simulink model "InnerOuter_Sim_newNav"  (Simulink 7.8)
settings: Solver=ode4  StartTime=0.0  StopTime=300  FixedStep=SampleT  RelTol=1e-3
InitFcn:
  | clc
  | innerOuterInit
values from neighbouring files (symbols this model uses):
  apSampleTime = 0.01    [innerOuterInit.m]
  SampleT = 0.005    [innerOuterInit.m]
  T = 0.01    [innerOuterInit.m]
undefined symbols (not defined in the file or in its folder): A1, Apolar, baseHeight, BasePoint, baseTemp, CD0, chord, CL0, CLa, CLa_dot, Clb, ClDa, CLDe, CLDf, ClDr, clock, Clp, CLq, Clr, Cm0, Cma, CmDe, CmDf, Cmq, Cnb, CnDa, CnDr, Cnp, Cnr, compensatorOn, CYb, CYDr, da_failamp, da_failbias, da_failper, daL_fail, daR_fail, deg, DiscIntNeverNeededParam, dr_fail, dr_failamp, dr_failbias, dr_failper, Earth, elarm, Euler_0, F, gaind, Init_onlyOnce, Init_Reset, ISA_g, Ixx, Iyy, Izz, L1OF, lapseRate, Light, mass, MIL, MinThK ... (+21)
libraries: simulink x69, aerolibconvert2 x19, SLUGS_Library x10, aerolibactuator x5, aerolibobsolete x3, dspmtrx3 x3, aerolibwind2 x2, aerolibtransform2 x1, aerolibatmos2 x1, dsPICdrivers x1
(part 1 of 3)
CloseFcn:
  | rtwprivate ssgencode ModelCloseRequest AttitudeComplementary
settings Model: Creator=ASL_Lab  LastModifiedBy=User  BufferReuse=off
settings OptimizationCC: BlockReduction=off  ConditionallyExecuteInputs=off  OptimizeBlockIOStorage=off  BufferReuse=off  ExpressionFolding=off  LocalBlockOutputs=off  InitFltsAndDblsToZero=on
settings DebuggingCC: ConsistencyChecking=warning  AlgebraicLoopMsg=error  SaveWithParameterizedLinksMsg=none  MultiTaskDSMMsg=warning  MultiTaskCondExecSysMsg=none  FcnCallInpInsideContextMsg=Use local settings  ModelReferenceExtraNoncontSigs=warning  StrictBusMsg=None
settings HardwareCC: TargetHWDeviceType=32-bit Generic
settings SFSimCC: SimParseCustomCode=off
settings RTWCC: IncludeERTFirstTime=on
settings GRTTargetCC: TargetFcnLib=ansi_tfl_tmw.mat

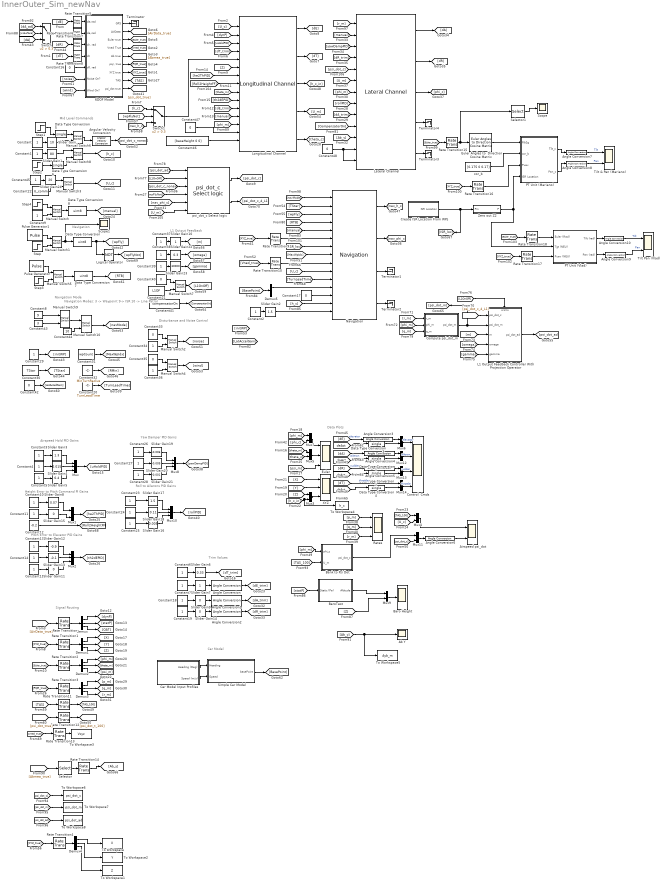
== system InnerOuter_Sim_newNav ==
  note: Mid Level Commands
  note: Trim Values
  note: Signal Routing
  note: Airspeed Hold PID Gains
  note: Height Error to Pitch Command PI Gains
  note: Pitch Error to Elevator PID Gains
  note: Data Plots
  note: Yaw Damper PID Gains
  note: Roll to Ailerons PID Gains
  note: Navigation
  note: Disturbance and Noise Control
  note: L1 Output Feedback
  note: Car Model
  note: Navigation Mode
  note: Navigation Modes:
      | 3 -> Waypoint
      | 9-> ISR
      | 10 -> Line Patrol
  6DOF Model : Subsystem
  Ab Y : Scope
      settings: TimeRange=140  YMin=-3  YMax=3  SaveName=ScopeData9
  Airspeed psi_dot : Scope  NumInputPorts=2
      settings: TimeRange=125  YMin=14.91~-37.5  YMax=15.05~5  SaveName=AirspeedPsiDot
  Angle Conversion : aerolibconvert2/Angle Conversion  IU=deg  OU=rad
  Angle Conversion1 : aerolibconvert2/Angle Conversion  IU=deg  OU=rad
  Angle Conversion{3..10} (8 alike) : aerolibconvert2/Angle Conversion  IU=rad  OU=deg
  Angle Conversion2 : aerolibconvert2/Angle Conversion  IU=deg  OU=rad
  Angular Velocity Conversion : aerolibconvert2/Angular Velocity Conversion  IU=deg/s  OU=rad/s
  Bank to Psi Dot : Subsystem  AncestorBlock=SLUGS_Library/Navigation/Bank to Psi Dot
  Baro Height : Scope
      settings: TimeRange=350  YMin=-1500  YMax=700  SaveName=AirspeedPsiDot1
  BaroTest : Subsystem
  Car Model Input Profiles : Subsystem  Tag=STV Subsys  LoadFcn=sigbuilder_block('load');  StartFcn=sigbuilder_block('start');  StopFcn=sigbuilder_block('stop');  ClipboardFcn=sigbuilder_block('clipboard');  mask(Sigbuilder block){}
      mask help: Sigbuilder GUI
      mask init:
      | if ~strcmp(get_param(bdroot(gcbh),'SimulationStatus'),'stopped') tuvar = sigbuilder_block('maskInit'); end
      settings: CopyFcn=sigbuilder_block('copy');  DeleteFcn=sigbuilder_block('delete');  ModelCloseFcn=sigbuilder_block('modelClose');  PreSaveFcn=sigbuilder_block('preSave');  NameChangeFcn=sigbuilder_block('namechange');  OpenFcn=sigbuilder_block('open',[437.25 199.5 550.5 399.75 ]);  CloseFcn=sigbuilder_block('close');
      mask Display: plot(0,0,100,100,[10,10,40,40,10],[80,20,20,80,80],[40,10],[50,50], [40,27,10],[65,72,56],[40,25,25,10],[28,28,43,43]);
  Compute psi_dot_m : Subsystem
  Constant{,1..7,10..11,13..15,18..19,23..28,37..39,45} (25 alike) : Constant  OutDataTypeStr=single  SampleTime=apSampleTime
  Constant12 : Constant  Value=-0.2  OutDataTypeStr=single  SampleTime=apSampleTime
  Constant16 : Constant  Value=0
  Constant{17,40,47..48} (4 alike) : Constant  Value=0  OutDataTypeStr=uint8  SampleTime=apSampleTime
  Constant20 : Constant  Value=TurnLeadTime  SampleTime=apSampleTime
  Constant21 : Constant  Value=L1OF  OutDataTypeStr=single  SampleTime=apSampleTime
  Constant22 : Constant  Value=U_comm  SampleTime=apSampleTime
  Constant29 : Constant  OutDataTypeStr=uint8  SampleTime=apSampleTime
  Constant30 : Constant  Value=TStar  OutDataTypeStr=single  SampleTime=apSampleTime
  Constant31 : Constant  Value=wpCount  OutDataTypeStr=uint8  SampleTime=apSampleTime
  Constant32 : Constant  Value=MinTurnRadius  SampleTime=apSampleTime
  Constant33 : Constant  Value=0  SampleTime=SampleT
  Constant34 : Constant  SampleTime=SampleT
  Constant35 : Constant  Value=0  SampleTime=SampleT
  Constant36 : Constant  SampleTime=SampleT
  Constant41 : Constant  Value=compensatorOn  SampleTime=apSampleTime
  Constant42 : Constant  Value=0  SampleTime=apSampleTime
  Constant43 : Constant  Value=3  OutDataTypeStr=uint8  SampleTime=apSampleTime
  Constant44 : Constant  Value=10  OutDataTypeStr=uint8  SampleTime=apSampleTime
  Constant46 : Constant  Value=[baseHeight 0 0]  OutDataTypeStr=single
  Constant8 : Constant  Value=9  OutDataTypeStr=uint8  SampleTime=apSampleTime
  Constant9 : Constant  OutDataTypeStr=uint8  SampleTime=apSampleTime
  Control  Cmds : Scope  NumInputPorts=4
      settings: TickLabels=on  TimeRange=100  YMin=-2~-10~-11~0.225  YMax=3.5~17.5~1~0.425  SaveName=ctrlCmds
  Create ISR Location From WPs : Subsystem
  Data Type Conversion : DataTypeConversion  OutDataTypeStr=uint8
  Data Type Conversion{1..6} (6 alike) : DataTypeConversion  OutDataTypeStr=single
  Data Type Conversion7 : DataTypeConversion  OutDataTypeStr=uint8
  Data Type Conversion8 : DataTypeConversion  OutDataTypeStr=uint8
  Demux{,1..4} (5 alike) : Demux  Outputs=3
  Demux5 : Demux  Outputs=[2 1]
  Euler : Scope  NumInputPorts=3
      settings: TimeRange=100  YMin=-0.4~-0.02~0  YMax=1~0.06~7  SaveName=EulerData  DataFormat=Structure
  Euler Angles to  Direction Cosine Matrix : aerolibobsolete/Euler Angles to  Direction Cosine Matrix
  L1 Output Feedback Controller With  Projection Operator : Subsystem  TreatAsAtomicUnit=on
  Lateral Channel : SLUGS_Library/Control Blocks/Lateral Channel
  Logical Operator : Logic  Operator=NOT  AllPortsSameDT=off  OutDataTypeStr=boolean
  Longitudinal Channel : SLUGS_Library/Control Blocks/Longitudinal Channel
  Manual Switch{,2,4,7..8,10} (6 alike) : simulink/Signal Routing/Manual Switch  sw=1  action=0  varsize=off
  Manual Switch{1,3,5..6,9} (5 alike) : simulink/Signal Routing/Manual Switch  sw=0  action=0  varsize=off
  Mux{,2,8,10} (4 alike) : Mux  Inputs=3
  Mux{1,3..7,9,11..14} (11 alike) : Mux  Inputs=2
  Navigation : SLUGS_Library/Navigation/Navigation
  PT Unit (Mariano) : Subsystem  TreatAsAtomicUnit=on  SystemSampleTime=0.01
  "PT Unit (Vlad) " : Subsystem
  Pulse Generator : DiscretePulseGenerator  Period=200*100  PulseWidth=30*100  PhaseDelay=120*100  SampleTime=0.01
  Pulse Generator1 : DiscretePulseGenerator  Period=70*100  PulseWidth=45*100  PhaseDelay=0*100  SampleTime=0.01
  Rate Transition{,1..4,9..18} (15 alike) : RateTransition  OutPortSampleTime=apSampleTime
  Rate Transition{5..8} (4 alike) : RateTransition  OutPortSampleTime=SampleT
  Rates : Scope  NumInputPorts=3
      settings: TimeRange=300  YMin=-0.75~-1.5~-0.3  YMax=1~1.5~0.7  SaveName=ScopeData3
  Scope : Scope
      settings: YMin=5.2  YMax=6.3  SaveName=ScopeData2
  Scope1 : Scope
      settings: TimeRange=400  YMin=0.95  YMax=1.05  SaveName=ScopeData10
  Selector : Selector  InputPortWidth=3  IndexOptions=Index vector (dialog)  Indices=[2]  OutputSizes=1
  Selector1 : Selector  InputPortWidth=3  IndexOptions=Index vector (dialog)  Indices=[3]  OutputSizes=1
  Simple Car Model : Subsystem
  Slider Gain : simulink/Math Operations/Slider Gain  low=-18  gain=10  high=18
  Slider Gain1 : simulink/Math Operations/Slider Gain  low=0  gain=80  high=800
  Slider Gain10 : simulink/Math Operations/Slider Gain  low=0  gain=1  high=10
  Slider Gain11 : simulink/Math Operations/Slider Gain  low=-0.1  gain=0  high=0
  Slider Gain12 : simulink/Math Operations/Slider Gain  low=-2  gain=-0.9  high=0.3
  Slider Gain13 : simulink/Math Operations/Slider Gain  low=-0.1  gain=-0.1  high=0
  Slider Gain14 : simulink/Math Operations/Slider Gain  low=-10  gain=0  high=10
  Slider Gain15 : simulink/Math Operations/Slider Gain  low=-20  gain=0  high=20
  Slider Gain16 : simulink/Math Operations/Slider Gain  low=-0.1  gain=0.005  high=0.1
  Slider Gain17 : simulink/Math Operations/Slider Gain  low=-0.1  gain=1.5  high=5
  Slider Gain18 : simulink/Math Operations/Slider Gain  low=0  gain=0.11  high=2
  Slider Gain19 : simulink/Math Operations/Slider Gain  low=-20  gain=-0.006  high=20
  Slider Gain2 : simulink/Math Operations/Slider Gain  low=0  gain=1.5  high=2
  Slider Gain20 : simulink/Math Operations/Slider Gain  low=-20  gain=-0.009  high=20
  Slider Gain21 : simulink/Math Operations/Slider Gain  low=-20  gain=-0.001  high=20
  Slider Gain22 : simulink/Math Operations/Slider Gain  low=0  gain=0.3  high=5
  Slider Gain23 : simulink/Math Operations/Slider Gain  low=-50000  gain=30000  high=50000
  Slider Gain24 : simulink/Math Operations/Slider Gain  low=0  gain=20  high=50
  Slider Gain3 : simulink/Math Operations/Slider Gain  low=0  gain=1.3  high=4.5
  Slider Gain4 : simulink/Math Operations/Slider Gain  low=-20  gain=0.015  high=20
  Slider Gain5 : simulink/Math Operations/Slider Gain  low=-20  gain=0.4  high=20
  Slider Gain6 : simulink/Math Operations/Slider Gain  low=0.1  gain=0.33  high=1
  Slider Gain7 : simulink/Math Operations/Slider Gain  low=-10  gain=1  high=10
  Slider Gain8 : simulink/Math Operations/Slider Gain  low=-20  gain=0.07  high=20
  Slider Gain9 : simulink/Math Operations/Slider Gain  low=-10  gain=0  high=10
  Step : Step  Time=0.01  SampleTime=0.01
  Step1 : Step  Time=10  After=5  SampleTime=0.01
  Step2 : Step  Time=10  Before=Pos_0(3)  After=500  SampleTime=0.01
  Step3 : Step  Time=1500  SampleTime=0.01
  Step4 : Step  Time=0.01  Before=1  After=0  SampleTime=0.01
  Switch : Switch  Criteria=u2 > Threshold  Threshold=0.3  OutDataTypeStr=Inherit: Inherit via back propagation  SampleTime=apSampleTime  InputSameDT=on
  Switch1 : Switch  Criteria=u2 > Threshold  Threshold=0.3  OutDataTypeStr=Inherit: Inherit via back propagation  InputSameDT=on
  Terminator{,1..4} (5 alike) : Terminator
  Tilt & Pan (Mariano) : Scope  NumInputPorts=2
      settings: TimeRange=125  YMin=60~-90  YMax=90~90  SaveName=AirspeedPsiDot2
  Tilt Pan (Vlad) : Scope  NumInputPorts=2
      settings: TimeRange=125  YMin=-100~-90  YMax=100~-50  SaveName=AirspeedPsiDot3
  To Workspace : ToWorkspace  VariableName=X  SampleTime=-1  SaveFormat=Array
  To Workspace1 : ToWorkspace  VariableName=Z  SampleTime=-1  SaveFormat=Array
  To Workspace2 : ToWorkspace  VariableName=Y  SampleTime=-1  SaveFormat=Array
  To Workspace3 : ToWorkspace  VariableName=Vxyz  SampleTime=-1  SaveFormat=Array
  To Workspace4 : ToWorkspace  VariableName=h_c  SampleTime=-1  SaveFormat=Array
  To Workspace5 : ToWorkspace  VariableName=Ayb_m  SampleTime=.01  SaveFormat=Array
  To Workspace6 : ToWorkspace  VariableName=psi_dot_c  SampleTime=.01  SaveFormat=Array
  To Workspace7 : ToWorkspace  VariableName=psi_dot_m  SampleTime=.01  SaveFormat=Array
  To Workspace8 : ToWorkspace  VariableName=psi_dot_ad  SampleTime=.01  SaveFormat=Array
  XYZ : Scope  NumInputPorts=3
      settings: TimeRange=125  YMin=-250~-200~180  YMax=100~200~230
  Zero out Z2 : MATLAB Function  TreatAsAtomicUnit=on
  cor_b : Constant  Value=[0.175 0 0.17]  OutDataTypeStr=single
  psi_dot_c Select logic : SLUGS_Library/Control Blocks/psi_dot_c Select logic
  wires:
  6DOF Model/7(XYZ true) -> [XYZ_true]
  6DOF Model/4(Vned True) -> [Vned_true]
  6DOF Model/5(Ab true) -> [Abmea_true]
  6DOF Model/6("pqr, true") -> [PQR_true]
  6DOF Model/3(Euler true) -> [Euler_true]
  6DOF Model/2(AirData) -> [AirData_true]
  Constant/1 -> Slider Gain/1
  Constant1/1 -> Slider Gain1/1
  ? -> ?
  Angular Velocity Conversion/1 -> [psi_dot_c_nonav]
  [AirData_true] -> Rate Transition/1
  Demux/1 -> [dynP]
  Demux/2 -> [statP]
  Demux/3 -> [OAT]
  Constant3/1 -> Slider Gain3/1
  Constant4/1 -> Slider Gain4/1
  Constant5/1 -> Slider Gain5/1
  Slider Gain4/1 -> Mux/2
  Slider Gain3/1 -> Mux/1
  Slider Gain5/1 -> Mux/3
  Mux/1 -> [uHoldPID]
  Constant6/1 -> Slider Gain6/1
  Slider Gain6/1 -> [dT_trim]
  [XYZ_true] -> Rate Transition1/1
  Demux1/1 -> [X]
  Demux1/2 -> [Y]
  Demux1/3 -> [Z]
  [Euler_true] -> Rate Transition2/1
  Demux2/1 -> [phi_m]
  Demux2/2 -> [theta_m]
  Demux2/3 -> [psi_m]
  Constant7/1 -> Slider Gain7/1
  Slider Gain7/1 -> Angle Conversion/1
  Angle Conversion/1 -> [dE_trim]
  Step4/1 -> Manual Switch/1
  Constant9/1 -> Manual Switch/2
  Manual Switch/1 -> Data Type Conversion8/1
  Constant10/1 -> Slider Gain8/1
  Constant11/1 -> Slider Gain15/1
  Slider Gain8/1 -> Mux1/1
  Mux1/1 -> [he2ThPID]
  Constant13/1 -> Slider Gain12/1
  Constant14/1 -> Slider Gain13/1
  Constant15/1 -> Slider Gain11/1
  Slider Gain13/1 -> Mux2/2
  Slider Gain12/1 -> Mux2/1
  Slider Gain11/1 -> Mux2/3
  Mux2/1 -> [th2dEPID]
  Mux5/1 -> Euler/2
  [psi_m] -> Euler/3
  [X] -> XYZ/1
  [Y] -> XYZ/2
  Mux3/1 -> XYZ/3
  [Z] -> Mux3/1
  [h_c_in] -> Mux3/2, To Workspace4/1
  [dT] -> Rate Transition8/1
  [dE] -> Rate Transition5/1
  Mux4/1 -> Airspeed psi_dot/1
  6DOF Model/8(TAS) -> [TAS]
  [TAS_100] -> Mux4/1
  [U_c] -> Mux4/2
  [theta_c] -> Mux5/2
  [PQR_true] -> Rate Transition3/1
  Demux3/1 -> [p_m]
  Demux3/2 -> [q_m]
  Demux3/3 -> [r_m]
  Constant18/1 -> Slider Gain9/1
  Slider Gain9/1 -> Angle Conversion1/1
  Angle Conversion1/1 -> [dA_trim]
  Constant19/1 -> Slider Gain14/1
  Slider Gain14/1 -> Angle Conversion2/1
  Angle Conversion2/1 -> [dR_trim]
  [r_m] -> Rates/3
  [q_m] -> Rates/2
  [phi_m] -> Mux7/1
  [phi_c] -> Mux7/2
  Mux7/1 -> Euler/1
  Constant26/1 -> Slider Gain19/1
  Constant27/1 -> Slider Gain20/1
  Constant28/1 -> Slider Gain21/1
  Slider Gain20/1 -> Mux8/2
  Slider Gain19/1 -> Mux8/1
  Slider Gain21/1 -> Mux8/3
  Mux8/1 -> [yawDampPID]
  Constant23/1 -> Slider Gain17/1
  Constant24/1 -> Slider Gain18/1
  Constant25/1 -> Slider Gain16/1
  Slider Gain18/1 -> Mux10/2
  Slider Gain17/1 -> Mux10/1
  Slider Gain16/1 -> Mux10/3
  Mux10/1 -> [rollPID]
  Switch/1 -> Rate Transition6/1
  [dR] -> Rate Transition7/1
  Constant16/1 -> 6DOF Model/5("df, rad")
  Slider Gain15/1 -> Mux1/2
  Mux6/1 -> Control  Cmds/1  "elevator"
  Mux12/1 -> Control  Cmds/2  "aileron"
  [theta_m] -> Mux5/1
  6DOF Model/9(psi_dot true) -> [psi_dot_true]
  Bank to Psi Dot/1(psi_dot_c) -> Mux11/1
  [psi_dot_c] -> Mux11/2
  Mux11/1 -> Angle Conversion6/1
  [p_m] -> Rates/1
  Pulse Generator1/1 -> Manual Switch1/1
  Step/1 -> Manual Switch1/2
  Manual Switch1/1 -> Data Type Conversion/1, Scope1/1
  Constant29/1 -> [initWP]
  Navigation/2 -> [nav_phi_c]
  [XYZ_true] -> Rate Transition9/1
  Constant30/1 -> [TStar]
  Constant31/1 -> [MaxWpIdx]
  [Vned_true] -> Rate Transition10/1
  [XYZ_true] -> Rate Transition4/1
  Demux4/1 -> To Workspace/1
  Demux4/2 -> To Workspace2/1
  Demux4/3 -> To Workspace1/1
  Navigation/1 -> [nav_h_c]
  Rate Transition/1 -> Demux/1
  Rate Transition1/1 -> Demux1/1
  Rate Transition2/1 -> Demux2/1
  Rate Transition3/1 -> Demux3/1
  Rate Transition4/1 -> Demux4/1
  [TAS] -> Rate Transition11/1
  Rate Transition11/1 -> [TAS_100]
  [psi_dot_true] -> Rate Transition12/1
  Rate Transition12/1 -> [psi_dot_t_100]
  Constant33/1 -> Manual Switch2/1
  Constant34/1 -> Manual Switch2/2
  Manual Switch2/1 -> [noise]
  [noise] -> 6DOF Model/6(Noise On?)
  Constant32/1 -> [RMin]
  6DOF Model/1(GPS) -> Terminator/1
  Slider Gain24/1 -> Manual Switch3/1
  Manual Switch3/1 -> [U_c]
  Constant22/1 -> Manual Switch3/2
  [dE] -> Angle Conversion3/1  "elevator"
  [deAct] -> Data Type Conversion3/1
  [dA] -> Angle Conversion4/1  "aileron"
  [daAct] -> Data Type Conversion1/1
  Mux13/1 -> Control  Cmds/3  "rudder"
  [dR] -> Angle Conversion5/1  "rudder"
  [drAct] -> Data Type Conversion2/1
  Mux14/1 -> Control  Cmds/4  "throttle"
  [dT] -> Mux14/1  "throttle"
  [dtAct] -> Data Type Conversion4/1
  Constant35/1 -> Manual Switch4/1
  Constant36/1 -> Manual Switch4/2
  Manual Switch4/1 -> [wind]
  [wind] -> 6DOF Model/7(Wind On?)
  Data Type Conversion/1 -> [wpFly], Logical Operator/1
  Data Type Conversion3/1 -> Mux6/2
  Data Type Conversion1/1 -> Mux12/2
  Data Type Conversion2/1 -> Mux13/2
  Data Type Conversion4/1 -> Mux14/2
  Rate Transition5/1 -> 6DOF Model/1(de,rad)
  Rate Transition8/1 -> 6DOF Model/4(dt)
  Rate Transition6/1 -> 6DOF Model/2(da,rad)
  Rate Transition7/1 -> 6DOF Model/3("dr, rad")
  Rate Transition13/1 -> To Workspace3/1
  [Vned_true] -> Rate Transition13/1
  Manual Switch6/1 -> Angular Velocity Conversion/1
  Slider Gain/1 -> Manual Switch6/2
  Step1/1 -> Data Type Conversion5/1
  Data Type Conversion5/1 -> Manual Switch6/1
  [psi_dot_c_4_L1] -> L1 Output Feedback Controller With  Projection Operator/1(psi_dot_c)
  L1 Output Feedback Controller With  Projection Operator/1(psi_dot_ad) -> [psi_dot_ad]
  [phi_m] -> Compute psi_dot_m/2(phi_m)
  [r_m] -> Compute psi_dot_m/1(r_m)
  Constant37/1 -> Slider Gain10/1
  Slider Gain10/1 -> [m]
  Constant38/1 -> Slider Gain22/1
  Slider Gain22/1 -> [omega]
  Constant39/1 -> Slider Gain23/1
  Slider Gain23/1 -> [gamma]
  [m] -> L1 Output Feedback Controller With  Projection Operator/3(m)
  [omega] -> L1 Output Feedback Controller With  Projection Operator/4(omega)
  [gamma] -> L1 Output Feedback Controller With  Projection Operator/5(gamma)
  Constant40/1 -> Manual Switch7/1
  Constant21/1 -> Manual Switch7/2
  Manual Switch7/1 -> [L1OnOff]
  [L1OnOff] -> L1 Output Feedback Controller With  Projection Operator/Enable
  [q_m] -> Compute psi_dot_m/3(q_m)
  Compute psi_dot_m/1(psi_dot_m) -> L1 Output Feedback Controller With  Projection Operator/2(psi_dot_m), [psi_dot_m]
  Angle Conversion3/1 -> Mux6/1
  Angle Conversion4/1 -> Mux12/1
  Angle Conversion5/1 -> Mux13/1
  [dA] -> Switch/3
  [dA_ad] -> Switch/1
  [L1Surface] -> Switch/2
  Constant41/1 -> [CompensatorOn]
  Manual Switch8/1 -> [h_c]
  Step2/1 -> Data Type Conversion6/1
  Slider Gain1/1 -> Manual Switch8/1
  Data Type Conversion6/1 -> Manual Switch8/2
  [statP] -> BaroTest/1(Static (Pa))
  Mux9/1 -> Baro Height/1
  [Z] -> Mux9/2
  BaroTest/1(Altitude) -> Mux9/1
  Selector/1 -> Rate Transition14/1
  [Abmea_true] -> Selector/1
  Rate Transition14/1 -> [Ab_y]
  [Ab_y] -> Ab Y/1, To Workspace5/1
  Angle Conversion6/1 -> Airspeed psi_dot/2
  [phi_m] -> Bank to Psi Dot/1(phi_c)
  [TAS_100] -> Bank to Psi Dot/2(U_m)
  [psi_dot_c] -> To Workspace6/1
  [psi_dot_m] -> To Workspace7/1
  [psi_dot_ad] -> To Workspace8/1
  Constant20/1 -> [TurnLeadTime]
  Constant42/1 -> [LatAccelGain]
  Pulse Generator/1 -> Manual Switch5/1
  Step3/1 -> Manual Switch5/2
  Manual Switch5/1 -> Data Type Conversion7/1
  Data Type Conversion7/1 -> [RTB]
  Demux5/1 -> Navigation/12
  Car Model Input Profiles/1(Heading (Deg)) -> Simple Car Model/1(Heading)
  Car Model Input Profiles/2(Speed (m/s)) -> Simple Car Model/2(Speed)
  Simple Car Model/1(basePoint) -> [BasePoint]
  [BasePoint] -> Demux5/1
  Constant43/1 -> Manual Switch9/2
  Constant8/1 -> Manual Switch9/1
  Manual Switch10/1 -> [navMode]
  Manual Switch9/1 -> Manual Switch10/1
  Constant44/1 -> Manual Switch10/2
  [Euler_true] -> Rate Transition15/1
  [XYZ_true] -> Rate Transition16/1
  Create ISR Location From WPs/1(ISR Location) -> [ISR_loc], Zero out Z2/1(Pin)
  Data Type Conversion8/1 -> [manual]
  Rate Transition15/1 -> Euler Angles to  Direction Cosine Matrix/1, Selector1/1
  Euler Angles to  Direction Cosine Matrix/1 -> PT Unit (Mariano)/1(Rb2g)
  cor_b/1 -> PT Unit (Mariano)/2(cor_b)
  Rate Transition16/1 -> PT Unit (Mariano)/3(Puav)
  PT Unit (Mariano)/1(Tilt_c) -> Angle Conversion7/1
  PT Unit (Mariano)/2(Pan_c) -> Angle Conversion8/1
  Angle Conversion7/1 -> Tilt & Pan (Mariano)/1  "Tilt"
  Angle Conversion8/1 -> Tilt & Pan (Mariano)/2  "Pan"
  Selector1/1 -> Scope/1
  Zero out Z2/1(P) -> PT Unit (Mariano)/4(ISR Location), "PT Unit (Vlad) "/2(Tgt (NEU))
  [XYZ_true] -> Rate Transition17/1
  Rate Transition17/1 -> "PT Unit (Vlad) "/3(Puav (NEU))
  [Euler_true] -> Rate Transition18/1
  Rate Transition18/1 -> "PT Unit (Vlad) "/1(Euler (Rad))
  "PT Unit (Vlad) "/2(Pan (rad)) -> Angle Conversion9/1
  "PT Unit (Vlad) "/1(Tilt (rad)) -> Angle Conversion10/1
  Angle Conversion10/1 -> Tilt Pan (Vlad)/1  "Tilt"
  Angle Conversion9/1 -> Tilt Pan (Vlad)/2  "Pan"
  [navMode] -> Navigation/1
  [TStar] -> Navigation/2
  [manual] -> Navigation/5
  [RTB] -> Navigation/4
  Rate Transition9/1 -> Navigation/6
  [ISR_loc] -> Navigation/7
  [MaxWpIdx] -> Navigation/8
  Rate Transition10/1 -> Navigation/9
  [U_c] -> Navigation/10
  [TurnLeadTime] -> Navigation/11
  Constant17/1 -> Navigation/13
  [h_c] -> Navigation/14
  Navigation/3 -> Terminator1/1
  Navigation/4 -> Terminator2/1
  Constant2/1 -> Slider Gain2/1
  Slider Gain2/1 -> Navigation/15
  Constant45/1 -> Slider Gain24/1
  [U_c] -> Longitudinal Channel/1
  [dynP] -> Longitudinal Channel/2
  [uHoldPID] -> Longitudinal Channel/3
  [dT_trim] -> Longitudinal Channel/4
  [Z] -> Longitudinal Channel/6
  [he2ThPID] -> Longitudinal Channel/7
  Longitudinal Channel/1 -> [dE]
  Longitudinal Channel/2 -> [dT]
  Longitudinal Channel/3 -> [h_c_in]
  Longitudinal Channel/4 -> [U_m]
  Longitudinal Channel/5 -> [theta_c]
  Constant46/1 -> Longitudinal Channel/15
  [theta_m] -> Longitudinal Channel/9
  [th2dEPID] -> Longitudinal Channel/10
  [dE_trim] -> Longitudinal Channel/11
  [manual] -> Longitudinal Channel/12
  [Roll2HeightFF] -> Longitudinal Channel/8
  Constant12/1 -> [Roll2HeightFF]
  [r_m] -> Lateral Channel/1
  [manual] -> Lateral Channel/2
  [yawDampPID] -> Lateral Channel/3
  [dR_trim] -> Lateral Channel/4
  [U_m] -> Lateral Channel/6
  [phi_m] -> Lateral Channel/7
  [rollPID] -> Lateral Channel/8
  [dA_trim] -> Lateral Channel/9
  Constant48/1 -> Lateral Channel/12, Lateral Channel/13
  Lateral Channel/1 -> [dA]
  Lateral Channel/2 -> [dR]
  Lateral Channel/3 -> [phi_c]
  Logical Operator/1 -> [wpFlyNot]
  [wpFly] -> Navigation/3
  [phi_m] -> Longitudinal Channel/13
  Constant47/1 -> Longitudinal Channel/14
  [wpFlyNot] -> Switch1/2
  [h_c] -> Switch1/1
  [nav_h_c] -> Switch1/3
  Switch1/1 -> Longitudinal Channel/5
  [psi_dot_ad] -> psi_dot_c Select logic/1
  [L1OnOff] -> psi_dot_c Select logic/2
  [psi_dot_c_nonav] -> psi_dot_c Select logic/3
  [wpFlyNot] -> psi_dot_c Select logic/4
  [nav_phi_c] -> psi_dot_c Select logic/5
  [U_m] -> psi_dot_c Select logic/6
  psi_dot_c Select logic/1 -> [psi_dot_c]
  psi_dot_c Select logic/2 -> [psi_dot_c_4_L1]
  [psi_dot_c] -> Lateral Channel/5
  [CompensatorOn] -> Lateral Channel/10
  [Ab_y] -> Lateral Channel/11
  Lateral Channel/4 -> Terminator4/1
  Lateral Channel/5 -> Terminator3/1

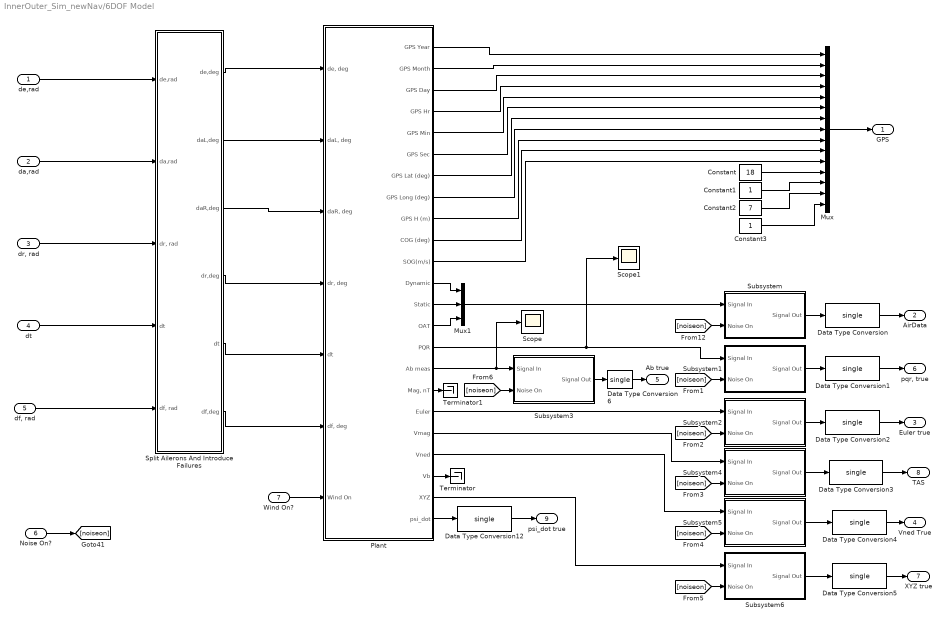
== system InnerOuter_Sim_newNav/6DOF Model ==
  de,rad : Inport
  da,rad : Inport  Port=2
  "dr, rad" : Inport  Port=3
  dt : Inport  Port=4
  "df, rad" : Inport  Port=5
  Noise On? : Inport  Port=6
  Wind On? : Inport  Port=7
  Constant : Constant  Value=18  SampleTime=SampleT
  Constant1 : Constant  SampleTime=SampleT
  Constant2 : Constant  Value=7  SampleTime=SampleT
  Constant3 : Constant  SampleTime=SampleT
  Data Type Conversion{,1..6,12} (8 alike) : DataTypeConversion  OutDataTypeStr=single
  Mux : Mux  Inputs=15
  Mux1 : Mux  Inputs=3
  Plant : Subsystem
  Scope : Scope
      settings: YMin=-13  YMax=1  SaveName=ScopeData5
  Scope1 : Scope
      settings: YMin=-0.05  YMax=0.04  SaveName=ScopeData6
  Split Ailerons And Introduce Failures : Subsystem
  Subsystem : Subsystem  mask{nv=[0.01 0.01 0.1], st=SampleT, ns=[132 564 987]}
      mask prompts: nv "Noise Variance"; st "Sample Time"; ns "Noise Seed"
  Subsystem1 : Subsystem  mask{nv=[0.001 0.001 0.001], st=SampleT, ns=[132 564 987]}
      mask prompts: nv "Noise Variance"; st "Sample Time"; ns "Noise Seed"
  Subsystem2 : Subsystem  mask{nv=[0.0001 0.00003 0.0001], st=SampleT, ns=[132 564 987]}
      mask prompts: nv "Noise Variance"; st "Sample Time"; ns "Noise Seed"
  Subsystem3 : Subsystem  mask{nv=[0.1 0.1 0.1], st=SampleT, ns=[132 564 987]}
      mask prompts: nv "Noise Variance"; st "Sample Time"; ns "Noise Seed"
  Subsystem4 : Subsystem  mask{nv=[0.01], st=SampleT, ns=[321564]}
      mask prompts: nv "Noise Variance"; st "Sample Time"; ns "Noise Seed"
  Subsystem5 : Subsystem  mask{nv=[0.01 0.01 0.01], st=SampleT, ns=[321564 6546 98798]}
      mask prompts: nv "Noise Variance"; st "Sample Time"; ns "Noise Seed"
  Subsystem6 : Subsystem  mask{nv=[0.05 0.05 0.07], st=SampleT, ns=[321564]}
      mask prompts: nv "Noise Variance"; st "Sample Time"; ns "Noise Seed"
  Terminator : Terminator
  Terminator1 : Terminator
  GPS : Outport
  AirData : Outport  Port=2
  Euler true : Outport  Port=3
  Vned True : Outport  Port=4
  Ab true : Outport  Port=5
  "pqr, true" : Outport  Port=6
  XYZ true : Outport  Port=7
  TAS : Outport  Port=8
  psi_dot true : Outport  Port=9
  wires:
  Mux/1 -> GPS/1
  Plant/1(GPS Year) -> Mux/1
  Plant/2(GPS Month) -> Mux/2
  Plant/3(GPS Day) -> Mux/3
  Plant/4(GPS Hr) -> Mux/4
  Plant/5(GPS Min) -> Mux/5
  Plant/6(GPS Sec) -> Mux/6
  Plant/7(GPS Lat (deg)) -> Mux/7
  Plant/8(GPS Long (deg)) -> Mux/8
  Plant/9(GPS H (m)) -> Mux/9
  Plant/10(COG (deg)) -> Mux/10
  Plant/11(SOG(m/s)) -> Mux/11
  Plant/12(Dynamic) -> Mux1/1
  Plant/13(Static) -> Mux1/2
  Plant/14(OAT) -> Mux1/3
  Mux1/1 -> Subsystem/1(Signal In)
  Constant/1 -> Mux/12
  Constant1/1 -> Mux/13
  Constant2/1 -> Mux/14
  Constant3/1 -> Mux/15
  Plant/23(psi_dot) -> Data Type Conversion12/1
  Noise On?/1 -> [noiseon]
  Subsystem/1(Signal Out) -> Data Type Conversion/1
  [noiseon] -> Subsystem/2(Noise On)
  [noiseon] -> Subsystem1/2(Noise On)
  [noiseon] -> Subsystem2/2(Noise On)
  [noiseon] -> Subsystem4/2(Noise On)
  [noiseon] -> Subsystem5/2(Noise On)
  [noiseon] -> Subsystem6/2(Noise On)
  [noiseon] -> Subsystem3/2(Noise On)
  Subsystem1/1(Signal Out) -> Data Type Conversion1/1
  Plant/15(PQR) -> Subsystem1/1(Signal In), Scope1/1
  Subsystem2/1(Signal Out) -> Data Type Conversion2/1
  Plant/18(Euler) -> Subsystem2/1(Signal In)
  Subsystem3/1(Signal Out) -> Data Type Conversion6/1
  Plant/16(Ab meas) -> Subsystem3/1(Signal In), Scope/1
  Subsystem4/1(Signal Out) -> Data Type Conversion3/1
  Plant/19(Vmag) -> Subsystem4/1(Signal In)
  Subsystem5/1(Signal Out) -> Data Type Conversion4/1
  Plant/20(Vned) -> Subsystem5/1(Signal In)
  Subsystem6/1(Signal Out) -> Data Type Conversion5/1
  Plant/22(XYZ) -> Subsystem6/1(Signal In)
  Plant/21(Vb) -> Terminator/1
  Plant/17("Mag, nT") -> Terminator1/1
  Split Ailerons And Introduce Failures/1(de,deg) -> Plant/1("de, deg")
  Split Ailerons And Introduce Failures/6(df,deg) -> Plant/6("df, deg")
  Split Ailerons And Introduce Failures/4(dr,deg) -> Plant/4("dr, deg")
  Split Ailerons And Introduce Failures/2(daL,deg) -> Plant/2("daL, deg")
  Wind On?/1 -> Plant/7(Wind On)
  Data Type Conversion/1 -> AirData/1
  Data Type Conversion1/1 -> "pqr, true"/1
  Data Type Conversion2/1 -> Euler true/1
  Data Type Conversion3/1 -> TAS/1
  Data Type Conversion4/1 -> Vned True/1
  Data Type Conversion5/1 -> XYZ true/1
  Data Type Conversion6/1 -> Ab true/1
  Data Type Conversion12/1 -> psi_dot true/1
  de,rad/1 -> Split Ailerons And Introduce Failures/1(de,rad)
  da,rad/1 -> Split Ailerons And Introduce Failures/2(da,rad)
  "dr, rad"/1 -> Split Ailerons And Introduce Failures/3("dr, rad")
  dt/1 -> Split Ailerons And Introduce Failures/4(dt)
  Split Ailerons And Introduce Failures/5("dt ") -> Plant/5(dt)
  "df, rad"/1 -> Split Ailerons And Introduce Failures/5("df, rad")
  Split Ailerons And Introduce Failures/3(daR,deg) -> Plant/3("daR, deg")

== system InnerOuter_Sim_newNav/Bank to Psi Dot ==
  phi_c : Inport
  U_m : Inport  Port=2
  Constant1 : Constant  Value=9.80665  OutDataTypeStr=single
  Divide : Product  Inputs=/*  OutDataTypeStr=single  SampleTime=apSampleTime
  Divide1 : Product  OutDataTypeStr=single  SampleTime=apSampleTime
  Subsystem8 : Subsystem  AncestorBlock=SLUGS_Library/Subsystem8
  negprotect : MATLAB Function  TreatAsAtomicUnit=on
  psi_dot_c : Outport
  wires:
  negprotect/1(zpVal) -> Divide/1
  Divide/1 -> Divide1/2
  phi_c/1 -> Subsystem8/1(x)
  Subsystem8/1(tan(x)) -> Divide1/1
  Divide1/1 -> psi_dot_c/1
  Constant1/1 -> Divide/2
  U_m/1 -> negprotect/1(val)

== system InnerOuter_Sim_newNav/BaroTest ==
  Static (Pa) : Inport
  Compute Barometric Height : Subsystem  mask{baseTemp=baseTemp, LapseRate=lapseRate}
      mask prompts: baseTemp "Base Station Temperature (K)"; LapseRate "Lapse Rate (C/ft)"
      mask help:
      | Produces Altitude in meters from Barometric Pressure in Pascals. Altitude is valid from MSL to 6000 ft.
      |
      | The method implemented here was developed by Ren Curry
  Constant1 : Constant  Value=baseHeight  OutDataTypeStr=single
  Enables/Disables the Computation of  initial Baro Bias : MATLAB Function  TreatAsAtomicUnit=on
  Initial Baro Bias : Subsystem  TreatAsAtomicUnit=on
  Sum1 : Sum  Inputs=++|  OutDataTypeStr=single
  Zero Out Height : Subsystem  TreatAsAtomicUnit=on
  Altitude : Outport
  wires:
  Compute Barometric Height/1("Altitude, m") -> Zero Out Height/2(Computed Height), Sum1/2
  Static (Pa)/1 -> Initial Baro Bias/1(Baro (Pa)), Compute Barometric Height/3(Baro (Pa))
  Enables/Disables the Computation of  initial Baro Bias/1(tOut) -> Initial Baro Bias/Enable, Zero Out Height/Enable
  Constant1/1 -> Compute Barometric Height/1(Base Height (m)), Zero Out Height/1(Base Height)
  Initial Baro Bias/1(Baro (Gnd)) -> Compute Barometric Height/2(Base Pressure (Pa))
  Zero Out Height/1(Height Offset) -> Sum1/1
  Sum1/1 -> Altitude/1

== system InnerOuter_Sim_newNav/Car Model Input Profiles ==
  Demux : Demux  Tag=STV Demux  Outputs=2
  FromWs : FromWorkspace  Tag=STV FromWs  VariableName=tuvar  SampleTime=0  SigBuilderData=DataTag0  VnvData=DataTag1
      SigBuilderData=|
      | common.afterFinalStr = 'Extrapolate'
      | common.sampleTime = 0
      | dataSet(1).timeRange = [0 400]
      | dataSet(1).name = 'High Speed'
      | dataSet(2).timeRange = [0 400]
      | dataSet(2).name = 'No Greater than the UAV'
      | dataSet(3).timeRange = [0 400]
      | dataSet(3).name = 'Constant Speed'
      | dataSet(4).timeRange = [0 1800]
      | dataSet(4).name = '1800 Run'
      | sbobj.Groups(1).Name = 'High Speed'
      | sbobj.Groups(1).Signals(1).Name = 'Heading (Deg)'
      | sbobj.Groups(1).Signals(1).XData = [0 25 25 50 50 75 75 100 100 125 125 150 150 175 175 200 200 225 225 250 250 275 275 300 300 325 325 350 350 375 375 400]
      | sbobj.Groups(1).Signals(1).YData = [90 90 -2 -4 90 90 -90 -90 -2 0 -90 -90 0 0 -90 -90 0 -2 88 88 90 90 0 0 -90 -88 -90 -90 2 2 -90 -90]
      | sbobj.Groups(1).Signals(2).Name = 'Speed (m/s)'
      | sbobj.Groups(1).Signals(2).XData = [0 50 100 150 200 250 300 350 400]
      | sbobj.Groups(1).Signals(2).YData = [0 14 18 12 5 9 12 18 18]
      | sbobj.Groups(1).TimeRange = [0 400]
      | sbobj.Groups(2).Name = 'No Greater than the UAV'
      | sbobj.Groups(2).Signals(1).Name = 'Heading (Deg)'
      | sbobj.Groups(2).Signals(1).XData = [0 25 25 50 50 75 75 100 100 125 125 150 150 175 175 200 200 225 225 250 250 275 275 300 300 325 325 350 350 375 375 400]
      | sbobj.Groups(2).Signals(1).YData = [90 90 -2 -4 90 90 -90 -90 -2 0 -90 -90 0 0 -90 -90 0 -2 88 88 90 90 0 0 -90 -88 -90 -90 2 2 -90 -90]
      | sbobj.Groups(2).Signals(2).Name = 'Speed (m/s)'
      | sbobj.Groups(2).Signals(2).XData = [0 50 100 150 200 250 300 350 400]
      | sbobj.Groups(2).Signals(2).YData = [5 14 -0.2 14.8 5 12.2 -0.2 15 15.2]
      | sbobj.Groups(2).TimeRange = [0 400]
      | sbobj.Groups(3).Name = 'Constant Speed'
      | sbobj.Groups(3).Signals(1).Name = 'Heading (Deg)'
      | sbobj.Groups(3).Signals(1).XData = [0 25 25 100 100 175 175 245 245 340 340 400]
      | sbobj.Groups(3).Signals(1).YData = [90 90 -2 -4 90 90 -90 -90 -2 0 -90 -90]
      | sbobj.Groups(3).Signals(2).Name = 'Speed (m/s)'
      | sbobj.Groups(3).Signals(2).XData = [0 50 100 150 200 250 300 350 400]
      | sbobj.Groups(3).Signals(2).YData = [10 10 9.98 9.99 9.99 10 10 10 10]
      | sbobj.Groups(3).TimeRange = [0 400]
      | sbobj.Groups(4).Name = '1800 Run'
      | sbobj.Groups(4).Signals(1).Name = 'Heading (Deg)'
      | sbobj.Groups(4).Signals(1).XData = [0 25 25 100 100 175 175 245 245 340 340 430 430 580 580 730 730 895 895 1105 1105 1325 1325 1515 1515 1725 1725 1800]
      | sbobj.Groups(4).Signals(1).YData = [90 90 -2 -4 90 90 -90 -90 -2 0 -90 -90 0 0 -90 -90 0 -2 90 90 0 0 -90 -90 2 2 -90 -90]
      | sbobj.Groups(4).Signals(2).Name = 'Speed (m/s)'
      | sbobj.Groups(4).Signals(2).XData = [0 50 100 150 200 680 880 1260 1260 1800]
      | sbobj.Groups(4).Signals(2).YData = [10 10 9.98 9.99 14.2 14.4 24.4 23.2 22.2 10.22]
      | sbobj.Groups(4).TimeRange = [0 1800]
  Heading (Deg) : Outport  Tag=STV Outport
  Speed (m/s) : Outport  Tag=STV Outport  Port=2
  wires:
  Demux/1 -> Heading (Deg)/1
  FromWs/1 -> Demux/1
  Demux/2 -> Speed (m/s)/1

== system InnerOuter_Sim_newNav/Compute psi_dot_m ==
  r_m : Inport
  phi_m : Inport  Port=2
  q_m : Inport  Port=3
  Product : Product  SampleTime=apSampleTime  RndMeth=Zero
  Product1 : Product  SampleTime=apSampleTime  RndMeth=Zero
  Subtract : Sum  Inputs=2
  dsPIC_cos : SLUGS_Library/dsPIC_cos
  dsPIC_sin : SLUGS_Library/dsPIC_sin
  psi_dot_m : Outport
  wires:
  dsPIC_cos/1 -> Product/2
  dsPIC_sin/1 -> Product1/2
  Product/1 -> Subtract/1
  Product1/1 -> Subtract/2
  r_m/1 -> Product/1
  phi_m/1 -> dsPIC_sin/1, dsPIC_cos/1
  Subtract/1 -> psi_dot_m/1
  q_m/1 -> Product1/1

== system InnerOuter_Sim_newNav/Create ISR Location From WPs ==
  Counter Limited : simulink/Sources/Counter Limited  uplimit=4  tsamp=150
  Display : Display
  RTB4 : Constant  OutDataTypeStr=uint8
  Rate Transition17 : RateTransition  X0=4  OutPortSampleTime=0.01
  Sum : Sum  Inputs=|++
  get sim WP Coord from Index : Subsystem
  ISR Location : Outport
  wires:
  RTB4/1 -> Sum/1
  Sum/1 -> Rate Transition17/1
  Rate Transition17/1 -> Display/1, get sim WP Coord from Index/1(WP Idx)
  Counter Limited/1 -> Sum/2
  get sim WP Coord from Index/1(WP Coord) -> ISR Location/1

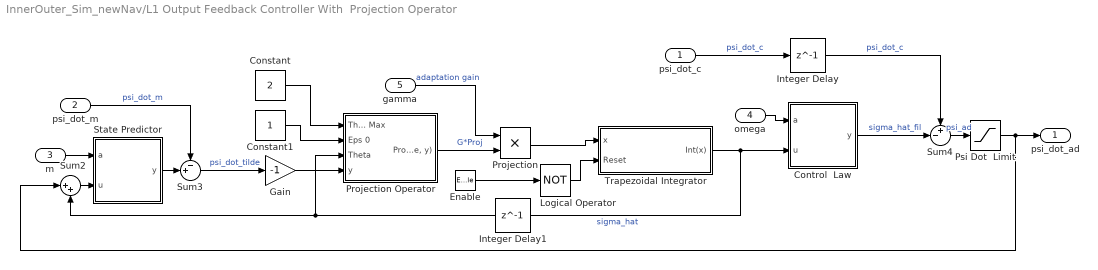
== system InnerOuter_Sim_newNav/L1 Output Feedback Controller With  Projection Operator ==
  psi_dot_c : Inport
  psi_dot_m : Inport  Port=2
  m : Inport  Port=3
  omega : Inport  Port=4
  gamma : Inport  Port=5
  Enable : EnablePort  ShowOutputPort=on
  Constant : Constant  Value=2  OutDataTypeStr=single
  Constant1 : Constant  OutDataTypeStr=single
  Control  Law : Subsystem
      mask Display:
      | droots([],'-a','a')
      | port_label('input',1,'a')
      | port_label('input',2,'u')
      | port_label('output',1,'y')
  Gain : Gain  Gain=-1  OutDataTypeStr=Inherit: Same as input
  Integer Delay : Delay  DelayLength=1  InputProcessing=Inherited  SampleTime=apSampleTime
  Integer Delay1 : Delay  DelayLength=1  InputProcessing=Inherited
  Logical Operator : Logic  Operator=NOT  AllPortsSameDT=off  OutDataTypeStr=uint(8)
  Projection : Product  SampleTime=apSampleTime  RndMeth=Zero
  Projection Operator : Subsystem
  Psi Dot  Limit : Saturate  UpperLimit=1  LowerLimit=-1  SampleTime=apSampleTime  OutDataTypeStr=single
  State Predictor : Subsystem
      mask Display:
      | droots([],'-a','a')
      | port_label('input',1,'a')
      | port_label('input',2,'u')
      | port_label('output',1,'y')
  Sum2 : Sum  Inputs=|++  SampleTime=apSampleTime
  Sum3 : Sum  Inputs=-+|
  Sum4 : Sum  Inputs=+-|  OutDataTypeStr=single  SampleTime=apSampleTime
  Trapezoidal Integrator : Subsystem  AncestorBlock=SLUGS_Library/Control Blocks/PID Controller w//Anti-Windup/Trapezoidal Integrator  mask{T=apSampleTime, upperLimit=2, lowerLimit=-2}
      mask prompts: T "Sample Time"; upperLimit "Upper Saturation"; lowerLimit "Lower Saturation"
  psi_dot_ad : Outport
  wires:
  Integer Delay1/1 -> Projection Operator/3(Theta), Sum2/2
  Constant1/1 -> Projection Operator/2(Eps 0)
  Constant/1 -> Projection Operator/1(Theta Max)
  Projection Operator/1("Proj(the, y)") -> Projection/2  "G*Proj"
  Sum4/1 -> Psi Dot  Limit/1  "psi_ad"
  Control  Law/1(y) -> Sum4/2  "sigma_hat_fil"
  omega/1 -> Control  Law/1(a)
  psi_dot_c/1 -> Integer Delay/1  "psi_dot_c"
  Trapezoidal Integrator/1(Int(x)) -> Control  Law/2(u), Integer Delay1/1  "sigma_hat"
  Projection/1 -> Trapezoidal Integrator/1(x)
  gamma/1 -> Projection/1  "adaptation gain"
  Sum3/1 -> Gain/1  "psi_dot_tilde"
  psi_dot_m/1 -> Sum3/1  "psi_dot_m"
  Sum2/1 -> State Predictor/2(u)
  m/1 -> State Predictor/1(a)
  Gain/1 -> Projection Operator/4(y)
  State Predictor/1(y) -> Sum3/2
  Integer Delay/1 -> Sum4/1  "psi_dot_c"
  Psi Dot  Limit/1 -> psi_dot_ad/1, Sum2/1
  Logical Operator/1 -> Trapezoidal Integrator/2(Reset)
  Enable/1 -> Logical Operator/1

== system InnerOuter_Sim_newNav/PT Unit (Mariano) ==
  Rb2g : Inport
  cor_b : Inport  Port=2
  Puav : Inport  Port=3
  ISR Location : Inport  Port=4
  Divide : Product  Inputs=*/
  Normalize : Product  Inputs=*/
  Product1 : Product  Multiplication=Matrix(*)  RndMeth=Zero
  Product2 : Product  Multiplication=Matrix(*)  RndMeth=Zero
  Subtract2 : Sum  Inputs=--+
  Transpose1 : dspmtrx3/Transpose  Hermitian=off  overflowFlag=off
  Vector Norm : SLUGS_Library/Vector Norm
  "[-90 90]" : Saturate  UpperLimit=1.5708  LowerLimit=-1.5708
  "[-90 90]1" : Saturate  UpperLimit=1.5708  LowerLimit=-1.5708
  "[a b c]" : Demux  Outputs=3
  dsPIC_asin : SLUGS_Library/dsPIC_asin
  dsPIC_atan : SLUGS_Library/dsPIC_atan
  Tilt_c : Outport
  Pan_c : Outport  Port=2
  wires:
  Rb2g/1 -> Transpose1/1, Product2/1  "Tbg"
  cor_b/1 -> Product1/2
  Vector Norm/1 -> Normalize/2
  Normalize/1 -> Product2/2
  Product2/1 -> "[a b c]"/1
  "[a b c]"/3 -> dsPIC_asin/1
  "[a b c]"/2 -> Divide/1
  "[a b c]"/1 -> Divide/2
  Divide/1 -> dsPIC_atan/1
  dsPIC_atan/1 -> "[-90 90]"/1
  Subtract2/1 -> Normalize/1, Vector Norm/1
  Transpose1/1 -> Product1/1
  "[-90 90]"/1 -> Pan_c/1
  "[-90 90]1"/1 -> Tilt_c/1
  dsPIC_asin/1 -> "[-90 90]1"/1
  ISR Location/1 -> Subtract2/3  "Xt"
  Puav/1 -> Subtract2/2  "Xac"
  Product1/1 -> Subtract2/1  "Tgb * cor_b"

== system InnerOuter_Sim_newNav/PT Unit (Vlad)  ==
  Euler (Rad) : Inport
  Tgt (NEU) : Inport  Port=2
  Puav (NEU) : Inport  Port=3
  Display1 : Display
  Divide : Product  Inputs=*/
  LPF the Euler and Construct Matrix : Subsystem
  Product1 : Product  Multiplication=Matrix(*)  RndMeth=Zero
  Subtract : Sum  Inputs=+-
  Trigonometric Function1 : Trigonometry  Operator=atan2
  Trigonometric Function2 : Trigonometry  Operator=asin
  Vector Norm : SLUGS_Library/Vector Norm
  "[-1 1]" : Saturate  UpperLimit=1  LowerLimit=-1
  "[-88 0]" : Saturate  UpperLimit=0  LowerLimit=-1.5708
  "[-98 98]" : Saturate  UpperLimit=1.7104  LowerLimit=-1.7104
  "[a b c]" : Demux  Outputs=3
  Tilt (rad) : Outport
  Pan (rad) : Outport  Port=2
  wires:
  Subtract/1 -> Product1/2  "Tgt_WR_UAV  (NEU)"
  LPF the Euler and Construct Matrix/1(Rfg2b) -> Product1/1
  "[a b c]"/2 -> Trigonometric Function1/1
  "[a b c]"/1 -> Trigonometric Function1/2
  Trigonometric Function1/1 -> "[-98 98]"/1
  Trigonometric Function2/1 -> "[-88 0]"/1, Display1/1
  Product1/1 -> "[a b c]"/1, Vector Norm/1
  "[-1 1]"/1 -> Trigonometric Function2/1
  "[a b c]"/3 -> Divide/1
  Vector Norm/1 -> Divide/2
  Divide/1 -> "[-1 1]"/1
  Euler (Rad)/1 -> LPF the Euler and Construct Matrix/1(Euler)
  "[-98 98]"/1 -> Pan (rad)/1
  Tgt (NEU)/1 -> Subtract/1
  "[-88 0]"/1 -> Tilt (rad)/1
  Puav (NEU)/1 -> Subtract/2

== system InnerOuter_Sim_newNav/Simple Car Model ==
  Heading : Inport
  Speed : Inport  Port=2
  Heading/Speed to Velocity : Subsystem
  Simple Car Model : Subsystem
  basePoint : Outport
  wires:
  Heading/Speed to Velocity/1(Velocity) -> Simple Car Model/1(Velocity)
  Heading/1 -> Heading/Speed to Velocity/1(Heading)
  Simple Car Model/1(p_cg) -> basePoint/1
  Speed/1 -> Heading/Speed to Velocity/2(Speed)

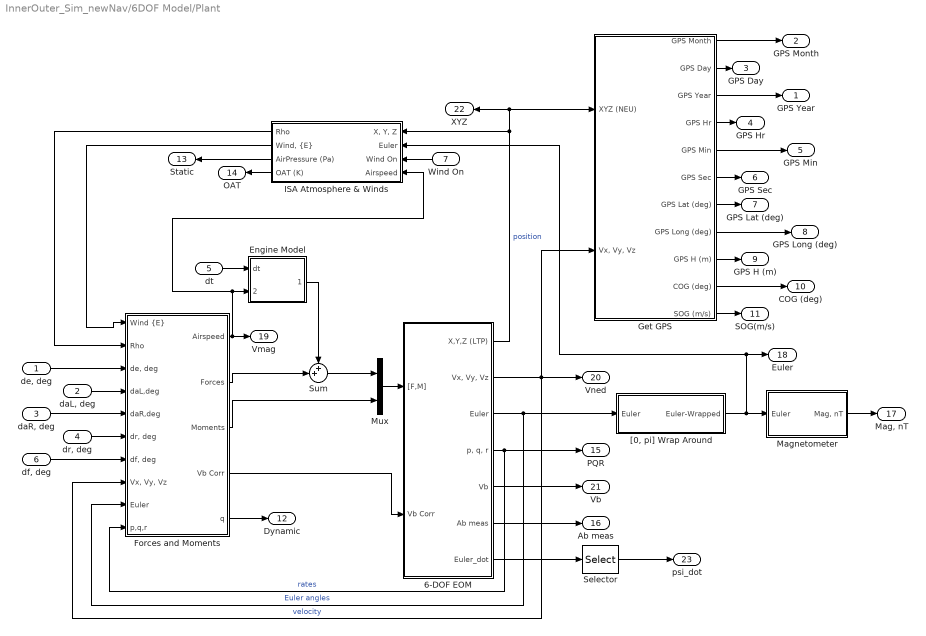
== system InnerOuter_Sim_newNav/6DOF Model/Plant ==
  "de, deg" : Inport
  "daL, deg" : Inport  Port=2
  "daR, deg" : Inport  Port=3
  "dr, deg" : Inport  Port=4
  dt : Inport  Port=5
  "df, deg" : Inport  Port=6
  Wind On : Inport  Port=7
  6-DOF EOM : Subsystem
  Engine Model : Subsystem
  Forces and Moments : Subsystem
  Get GPS : Subsystem
  ISA Atmosphere & Winds : Subsystem
  Magnetometer : Subsystem  mask{magField=[ 23143.6 5858.2 45511.9]}
      mask prompts: magField "Local Magnetic Field"
      mask help:
      | Simulates the Data from magnetometers with no noise.
      |
      | You can obtain data for the local magnetic field at:
      |
      | http://www.ngdc.noaa.gov/geomagmodels/IGRFWMM.jsp
  Mux : Mux  Inputs=2
  Selector : Selector  InputPortWidth=3  IndexOptions=Index vector (dialog)  Indices=[3]  OutputSizes=1
  Sum : Sum  Inputs=++|  SaturateOnIntegerOverflow=on
  "[0, pi] Wrap Around" : Subsystem
  GPS Year : Outport
  GPS Month : Outport  Port=2
  GPS Day : Outport  Port=3
  GPS Hr : Outport  Port=4
  GPS Min : Outport  Port=5
  GPS Sec : Outport  Port=6
  GPS Lat (deg) : Outport  Port=7
  GPS Long (deg) : Outport  Port=8
  GPS H (m) : Outport  Port=9
  COG (deg) : Outport  Port=10
  SOG(m/s) : Outport  Port=11
  Dynamic : Outport  Port=12
  Static : Outport  Port=13
  OAT : Outport  Port=14
  PQR : Outport  Port=15
  Ab meas : Outport  Port=16
  "Mag, nT" : Outport  Port=17
  Euler : Outport  Port=18
  Vmag : Outport  Port=19
  Vned : Outport  Port=20
  Vb : Outport  Port=21
  XYZ : Outport  Port=22
  psi_dot : Outport  Port=23
  wires:
  Get GPS/1(GPS Month) -> GPS Month/1
  Get GPS/2(GPS Day) -> GPS Day/1
  Get GPS/3(GPS Year) -> GPS Year/1
  Get GPS/4(GPS Hr) -> GPS Hr/1
  Get GPS/5(GPS Min) -> GPS Min/1
  Get GPS/6(GPS Sec) -> GPS Sec/1
  Get GPS/7(GPS Lat (deg)) -> GPS Lat (deg)/1
  Get GPS/8(GPS Long (deg)) -> GPS Long (deg)/1
  Get GPS/9(GPS H (m)) -> GPS H (m)/1
  6-DOF EOM/6(Ab meas) -> Ab meas/1
  Mux/1 -> 6-DOF EOM/1("[F,M]")
  6-DOF EOM/5(Vb) -> Vb/1
  Engine Model/1(Thrust) -> Sum/1
  Forces and Moments/5(q) -> Dynamic/1
  ISA Atmosphere & Winds/3(AirPressure (Pa)) -> Static/1
  Forces and Moments/1(Airspeed) -> Vmag/1, Engine Model/2(Vmag), ISA Atmosphere & Winds/4(Airspeed)
  ISA Atmosphere & Winds/2("Wind, {E}") -> Forces and Moments/1("Wind {E}")
  ISA Atmosphere & Winds/1(Rho) -> Forces and Moments/2(Rho)
  Forces and Moments/3(Moments) -> Mux/2
  Forces and Moments/2(Forces) -> Sum/2
  Sum/1 -> Mux/1
  Forces and Moments/4(Vb Corr) -> 6-DOF EOM/2(Vb Corr)
  6-DOF EOM/1(X,Y,Z (LTP)) -> ISA Atmosphere & Winds/1("X, Y, Z"), Get GPS/1(XYZ (NEU)), XYZ/1  "position"
  6-DOF EOM/2("Vx, Vy, Vz") -> Vned/1, Get GPS/2("Vx, Vy, Vz"), Forces and Moments/8("Vx, Vy, Vz ")  "velocity"
  6-DOF EOM/3(Euler) -> "[0, pi] Wrap Around"/1(Euler), Forces and Moments/9(Euler)  "Euler angles"
  6-DOF EOM/4("p, q, r") -> PQR/1, Forces and Moments/10(p,q,r)  "rates"
  dt/1 -> Engine Model/1(dt)
  "de, deg"/1 -> Forces and Moments/3("de, deg")
  "daL, deg"/1 -> Forces and Moments/4(daL,deg)
  "dr, deg"/1 -> Forces and Moments/6("dr, deg")
  "df, deg"/1 -> Forces and Moments/7("df, deg")
  "[0, pi] Wrap Around"/1(Euler-Wrapped) -> Magnetometer/1(Euler), Euler/1, ISA Atmosphere & Winds/2(Euler)
  Magnetometer/1("Mag, nT") -> "Mag, nT"/1
  Get GPS/10(COG (deg)) -> COG (deg)/1
  Get GPS/11(SOG (m/s)) -> SOG(m/s)/1
  ISA Atmosphere & Winds/4(OAT (K)) -> OAT/1
  6-DOF EOM/7(Euler_dot) -> Selector/1
  Selector/1 -> psi_dot/1
  Wind On/1 -> ISA Atmosphere & Winds/3(Wind On)
  "daR, deg"/1 -> Forces and Moments/5(daR,deg)

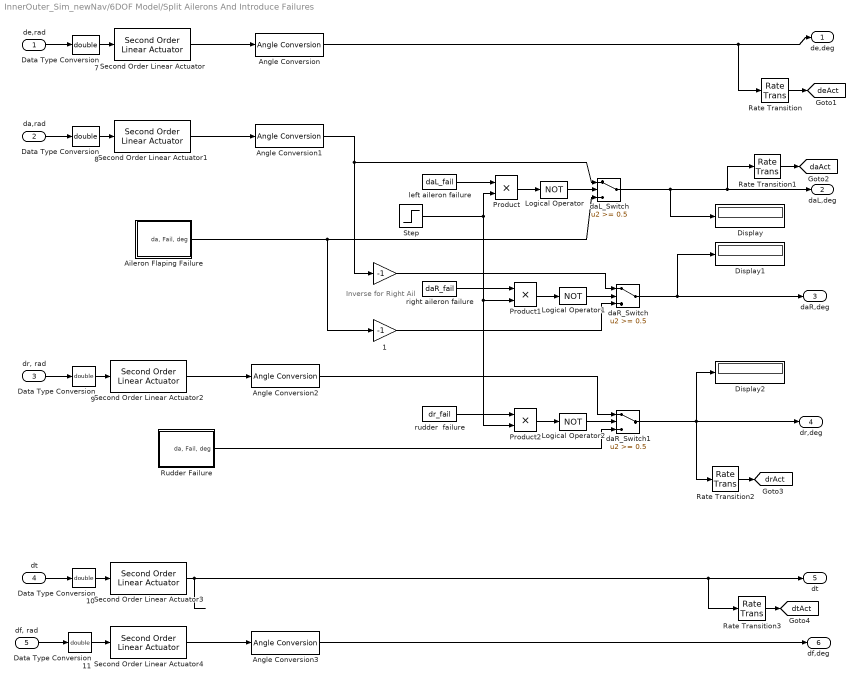
== system InnerOuter_Sim_newNav/6DOF Model/Split Ailerons And Introduce Failures ==
  note: Inverse
      | for Right
      | Ail
  de,rad : Inport
  da,rad : Inport  Port=2
  "dr, rad" : Inport  Port=3
  dt : Inport  Port=4
  "df, rad" : Inport  Port=5
  " " : Gain  Gain=-1  SaturateOnIntegerOverflow=on  OutDataTypeStr=Inherit: Same as input  ParamDataTypeStr=Inherit: Same as input
  " 1" : Gain  Gain=-1  SaturateOnIntegerOverflow=on  OutDataTypeStr=Inherit: Same as input  ParamDataTypeStr=Inherit: Same as input
  Aileron Flaping Failure : Subsystem
  Angle Conversion{,1..3} (4 alike) : aerolibconvert2/Angle Conversion  IU=rad  OU=deg
  Data Type Conversion{7..11} (5 alike) : DataTypeConversion  OutDataTypeStr=double
  Display : Display
  Display1 : Display
  Display2 : Display
  Logical Operator : Logic  Operator=NOT  AllPortsSameDT=off  OutDataTypeStr=boolean
  Logical Operator1 : Logic  Operator=NOT  AllPortsSameDT=off  OutDataTypeStr=boolean
  Logical Operator2 : Logic  Operator=NOT  AllPortsSameDT=off  OutDataTypeStr=boolean
  Product : Product  RndMeth=Zero
  Product1 : Product  RndMeth=Zero
  Product2 : Product  RndMeth=Zero
  Rate Transition{,1..3} (4 alike) : RateTransition  OutPortSampleTime=apSampleTime
  Rudder Failure : Subsystem
  Second Order Linear Actuator{,1..3} (4 alike) : aerolibactuator/Second Order Linear Actuator  wn_fin=15  z_fin=0.8  fin_act_0=0
  Second Order Linear Actuator4 : aerolibactuator/Second Order Linear Actuator  wn_fin=150  z_fin=0.7  fin_act_0=0
  Step : Step  Time=tfailure
  daL_Switch : Switch  Threshold=0.5
  daR_Switch : Switch  Threshold=0.5
  daR_Switch1 : Switch  Threshold=0.5
  left aileron failure : Constant  Value=daL_fail
  right aileron failure : Constant  Value=daR_fail
  rudder  failure : Constant  Value=dr_fail
  de,deg : Outport
  daL,deg : Outport  Port=2
  daR,deg : Outport  Port=3
  dr,deg : Outport  Port=4
  "dt " : Outport  Port=5
  df,deg : Outport  Port=6
  tag scope: daAct=global, deAct=global, drAct=global, dtAct=global
  wires:
  de,rad/1 -> Data Type Conversion7/1
  da,rad/1 -> Data Type Conversion8/1
  "dr, rad"/1 -> Data Type Conversion9/1
  dt/1 -> Data Type Conversion10/1
  "df, rad"/1 -> Data Type Conversion11/1
  Second Order Linear Actuator/1 -> Angle Conversion/1
  Second Order Linear Actuator1/1 -> Angle Conversion1/1
  Second Order Linear Actuator2/1 -> Angle Conversion2/1
  Second Order Linear Actuator3/1 -> "dt "/1, Rate Transition3/1
  Second Order Linear Actuator4/1 -> Angle Conversion3/1
  Rate Transition1/1 -> [daAct]
  Rate Transition2/1 -> [drAct]
  Rate Transition3/1 -> [dtAct]
  Data Type Conversion7/1 -> Second Order Linear Actuator/1
  Data Type Conversion8/1 -> Second Order Linear Actuator1/1
  Data Type Conversion9/1 -> Second Order Linear Actuator2/1
  Data Type Conversion10/1 -> Second Order Linear Actuator3/1
  Data Type Conversion11/1 -> Second Order Linear Actuator4/1
  Angle Conversion/1 -> de,deg/1, Rate Transition/1
  Angle Conversion1/1 -> daL_Switch/1, " "/1
  Angle Conversion2/1 -> daR_Switch1/1
  Angle Conversion3/1 -> df,deg/1
  left aileron failure/1 -> Product/1
  Aileron Flaping Failure/1("da, Fail, deg") -> daL_Switch/3, " 1"/1
  Product/1 -> Logical Operator/1
  Logical Operator/1 -> daL_Switch/2
  Step/1 -> Product/2, Product1/2, Product2/2
  daL_Switch/1 -> Display/1, daL,deg/1, Rate Transition1/1
  right aileron failure/1 -> Product1/1
  Product1/1 -> Logical Operator1/1
  Logical Operator1/1 -> daR_Switch/2
  " "/1 -> daR_Switch/1
  " 1"/1 -> daR_Switch/3
  daR_Switch/1 -> daR,deg/1, Display1/1
  rudder  failure/1 -> Product2/1
  Product2/1 -> Logical Operator2/1
  Logical Operator2/1 -> daR_Switch1/2
  daR_Switch1/1 -> dr,deg/1, Display2/1, Rate Transition2/1
  Rate Transition/1 -> [deAct]
  Rudder Failure/1("da, Fail, deg") -> daR_Switch1/3

== system InnerOuter_Sim_newNav/6DOF Model/Subsystem ==
  Signal In : Inport
  Noise On : Inport  Port=2
  Add : Sum
  Random Number : RandomNumber  Variance=nv  Seed=ns  SampleTime=st
  Signal1 : InportShadow  Port=1
  Switch : Switch  Threshold=0.3
  Signal Out : Outport
  wires:
  Random Number/1 -> Add/2
  Add/1 -> Switch/1
  Signal In/1 -> Add/1
  Noise On/1 -> Switch/2
  Switch/1 -> Signal Out/1
  Signal1/1 -> Switch/3

== system InnerOuter_Sim_newNav/6DOF Model/Subsystem1 ==
  Signal In : Inport
  Noise On : Inport  Port=2
  Add : Sum
  Random Number : RandomNumber  Variance=nv  Seed=ns  SampleTime=st
  Signal1 : InportShadow  Port=1
  Switch : Switch  Threshold=0.3
  Signal Out : Outport
  wires:
  Signal1/1 -> Switch/3
  Switch/1 -> Signal Out/1
  Noise On/1 -> Switch/2
  Signal In/1 -> Add/1
  Add/1 -> Switch/1
  Random Number/1 -> Add/2

== system InnerOuter_Sim_newNav/6DOF Model/Subsystem2 ==
  Signal In : Inport
  Noise On : Inport  Port=2
  Add : Sum
  Random Number : RandomNumber  Variance=nv  Seed=ns  SampleTime=st
  Signal1 : InportShadow  Port=1
  Switch : Switch  Threshold=0.3
  Signal Out : Outport
  wires:
  Random Number/1 -> Add/2
  Add/1 -> Switch/1
  Signal In/1 -> Add/1
  Noise On/1 -> Switch/2
  Switch/1 -> Signal Out/1
  Signal1/1 -> Switch/3

== system InnerOuter_Sim_newNav/6DOF Model/Subsystem3 ==
  Signal In : Inport
  Noise On : Inport  Port=2
  Add : Sum
  Random Number : RandomNumber  Variance=nv  Seed=ns  SampleTime=st
  Signal1 : InportShadow  Port=1
  Switch : Switch  Threshold=0.3
  Signal Out : Outport
  wires:
  Signal1/1 -> Switch/3
  Switch/1 -> Signal Out/1
  Noise On/1 -> Switch/2
  Signal In/1 -> Add/1
  Add/1 -> Switch/1
  Random Number/1 -> Add/2

== system InnerOuter_Sim_newNav/6DOF Model/Subsystem4 ==
  Signal In : Inport
  Noise On : Inport  Port=2
  Add : Sum
  Random Number : RandomNumber  Variance=nv  Seed=ns  SampleTime=st
  Signal1 : InportShadow  Port=1
  Switch : Switch  Threshold=0.3
  Signal Out : Outport
  wires:
  Signal1/1 -> Switch/3
  Switch/1 -> Signal Out/1
  Noise On/1 -> Switch/2
  Signal In/1 -> Add/1
  Add/1 -> Switch/1
  Random Number/1 -> Add/2

== system InnerOuter_Sim_newNav/6DOF Model/Subsystem5 ==
  Signal In : Inport
  Noise On : Inport  Port=2
  Add : Sum
  Random Number : RandomNumber  Variance=nv  Seed=ns  SampleTime=st
  Signal1 : InportShadow  Port=1
  Switch : Switch  Threshold=0.3
  Signal Out : Outport
  wires:
  Random Number/1 -> Add/2
  Add/1 -> Switch/1
  Signal In/1 -> Add/1
  Noise On/1 -> Switch/2
  Switch/1 -> Signal Out/1
  Signal1/1 -> Switch/3

== system InnerOuter_Sim_newNav/6DOF Model/Subsystem6 ==
  Signal In : Inport
  Noise On : Inport  Port=2
  Add : Sum
  Random Number : RandomNumber  Variance=nv  Seed=ns  SampleTime=st
  Signal1 : InportShadow  Port=1
  Switch : Switch  Threshold=0.3
  Signal Out : Outport
  wires:
  Signal1/1 -> Switch/3
  Switch/1 -> Signal Out/1
  Noise On/1 -> Switch/2
  Signal In/1 -> Add/1
  Add/1 -> Switch/1
  Random Number/1 -> Add/2

== system InnerOuter_Sim_newNav/Bank to Psi Dot/Subsystem8 ==
  x : Inport
  C Function Call1 : dsPICdrivers/OTHERS/C Function Call  Tag=dsPIC_dsPIC_CFunctionCall  FctUpdate=Output Function  fctName='myTan'  INPUT_SIZE=1  INPUT1=real32  INPUT2=--  INPUT3=--  OUTPUT_SIZE=1  OUTPUT1=real32  SampleTime=-1  InputType=[ 7 ]  OutputType=[ 7 ]  FctDeclaration=extern real32_T myTan(real32_T u1);  FctCall=%y1 = myTan(%u1);  OrderingInOutPopup=None  FctStart=None  FctStart_Name=Init_onlyOnce  FctStart_Declaration=inline extern void Init_onlyOnce();  FctStart_Call=Init_onlyOnce();  FctInit=None  FctInit_Name=Init_Reset  FctInit_Declaration=inline extern void Init_Reset();  FctInit_Call=Init_Reset();  PinDigitalInput=[]  PinDigitalOutput=[]  AnalogueInput=[]
  Environment Controller : simulink/Signal Routing/Environment Controller
  Trigonometric Function : Trigonometry  Operator=tan
  tan(x) : Outport
  wires:
  Environment Controller/1 -> tan(x)/1
  C Function Call1/1 -> Environment Controller/2
  Trigonometric Function/1 -> Environment Controller/1
  x/1 -> Trigonometric Function/1, C Function Call1/1
